simulink library "tether002_ul"  (R2020a)
settings: Solver=VariableStepAuto  StartTime=0.0  StopTime=10.0  RelTol=1e-3
values from neighbouring files (symbols this model uses):
  initNodePos = [INITIALLINE;INITIALLINE;INITIALLINE]    [tether002_ts.m]
  initNodeVel = [zeros(1,numNodes-2);zeros(1,numNodes-2);zeros(1,numNodes-2)]    [tether002_ts.m]
  numNodes = 11    [tether002_ts.m]
undefined symbols (not defined in the file or in its folder): TotoalNodes
libraries: powerlib_meascontrol x11, nodePosToLinkPos_ul x6, dspmtrx3 x4, sharedtransform x3, simulink_extras x2
(part 1 of 4)
settings Model: Creator=mitch  LastModifiedBy=mr-jo

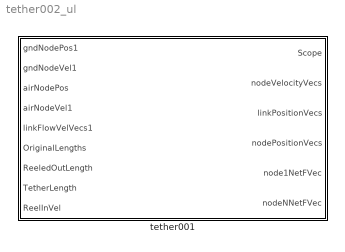
== system tether002_ul ==
  tether001 : Subsystem

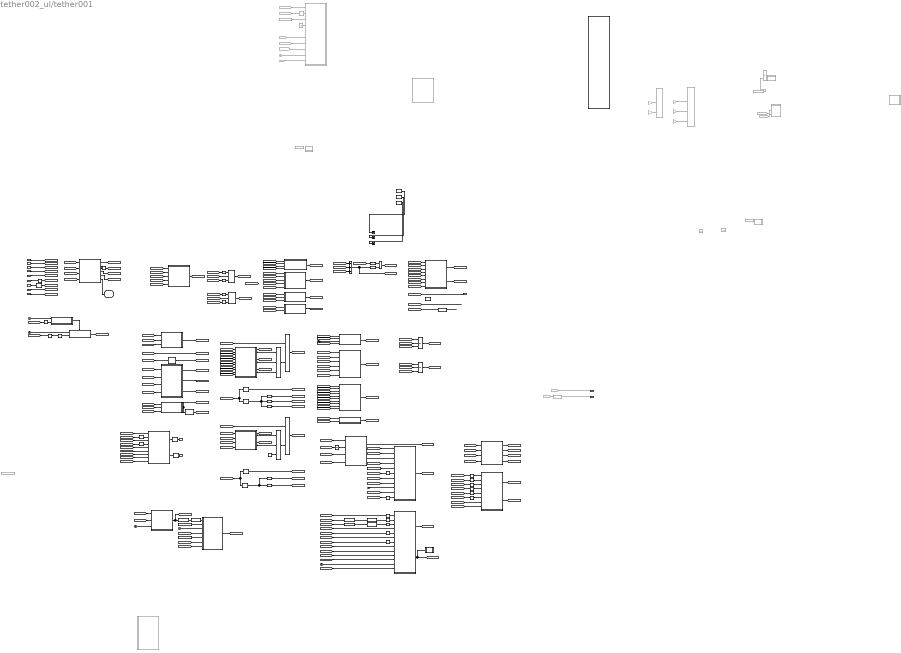
== system tether002_ul/tether001 ==
  note: "Dumbell" Edit
  gndNodePos1 : Inport
  gndNodeVel1 : Inport  Port=2
  airNodePos : Inport  Port=3
  airNodeVel1 : Inport  Port=4
  linkFlowVelVecs1 : Inport  Port=5
  OriginalLengths : Inport  Port=6
  ReeledOutLength : Inport  Port=7
  TetherLength : Inport  Port=8
  ReelInVel : Inport  Port=9
  Add4 : Sum  Inputs=3
  Clock{,1..2,4..7} (7 alike) : Clock
  Clock3 : Clock  Commented=on
  Constant : Constant  Value=0
  Constant1 : Constant  Commented=on  Value=[initNodeVel]
  Constant11 : Constant  Commented=on  Value=[initNodeVel,zeros(3,3)]
  Constant16 : Constant  Value=[initNodeVel,zeros(3,1)]
  Constant2 : Constant  Value=[initNodePos]
  Constant3 : Constant  Value=[numNodes]
  Constant7 : Constant  Commented=on  Value=[initNodePos]
  Direction Cosine Matrix to Rotation Angles : sharedtransform/Direction Cosine Matrix to Rotation Angles  rotationOrder=ZYX  aMode=aMode  action=None  tolerance=eps(2)
      settings: SourceProductBaseCode=AE,PW,MT,VE,VP
  Direction Cosine Matrix to Rotation Angles1 : sharedtransform/Direction Cosine Matrix to Rotation Angles  rotationOrder=ZYX  aMode=aMode  action=None  tolerance=eps(2)
      settings: SourceProductBaseCode=AE,PW,MT,VE,VP
  Direction Cosine Matrix to Rotation Angles2 : sharedtransform/Direction Cosine Matrix to Rotation Angles  rotationOrder=ZYX  aMode=aMode  action=None  tolerance=eps(2)
      settings: SourceProductBaseCode=AE,PW,MT,VE,VP
  First-Order Filter : powerlib_meascontrol/Filters/First-Order Filter  FilterType=Lowpass  Tc=10e-3  Ts=0  Initialize=on  Vac_Init=[0, 0, 60]  Vdc_Init=100  PlotResponse=off  FreqRange="[0,  200,  1]"
  First-Order Filter1 : powerlib_meascontrol/Filters/First-Order Filter  FilterType=Lowpass  Tc=.001  Ts=0  Initialize=on  Vac_Init=[0, 0, 60]  Vdc_Init=0  PlotResponse=off  FreqRange="[0,  200,  1]"
  First-Order Filter{2..4,7..8} (5 alike) : powerlib_meascontrol/Filters/First-Order Filter  FilterType=Lowpass  Tc=1  Ts=0  Initialize=on  Vac_Init=[0, 0, 60]  Vdc_Init=0  PlotResponse=off  FreqRange="[0,  200,  1]"
  First-Order Filter5 : powerlib_meascontrol/Filters/First-Order Filter  FilterType=Lowpass  Tc=10e-3  Ts=0  Initialize=on  Vac_Init=[0, 0, 60]  Vdc_Init=0  PlotResponse=off  FreqRange="[0,  200,  1]"
  First-Order Filter6 : powerlib_meascontrol/Filters/First-Order Filter  FilterType=Lowpass  Tc=10e-3  Ts=0  Initialize=on  Vac_Init=[0, 0, 60]  Vdc_Init=0  PlotResponse=off  FreqRange="[0,  200,  1]"
  From{1,105..106,113} (4 alike) : From  Commented=on  GotoTag=ActiveNodes
  From112 : From  Commented=on  GotoTag=gndNodePos
  From114 : From  Commented=on  GotoTag=OriginalLengths
  From119 : From  Commented=on  GotoTag=Ld
  From161 : From  Commented=on  GotoTag=nodeVel
  From165 : From  Commented=on  GotoTag=nodePos
  From27 : From  Commented=on  GotoTag=o_a_AO_O
  HowManyActive3 : MATLAB Function  TreatAsAtomicUnit=on
  Integrator1 : Integrator  ExternalReset=rising  InitialConditionSource=external
  Integrator8 : Integrator  ExternalReset=rising  InitialConditionSource=external
  Integrator9 : Integrator  Commented=on  InitialConditionSource=external
  MATLAB Function : MATLAB Function  Commented=on  TreatAsAtomicUnit=on
  MATLAB Function1 : MATLAB Function  Commented=on  TreatAsAtomicUnit=on
  MATLAB Function11 : MATLAB Function  Commented=on  TreatAsAtomicUnit=on
  MATLAB Function15 : MATLAB Function  Commented=on  TreatAsAtomicUnit=on
  MATLAB Function2 : MATLAB Function  TreatAsAtomicUnit=on
  MATLAB Function23 : MATLAB Function  TreatAsAtomicUnit=on
  MATLAB Function24 : MATLAB Function  TreatAsAtomicUnit=on
  MATLAB Function25 : MATLAB Function  TreatAsAtomicUnit=on
  MATLAB Function26 : MATLAB Function  Commented=on  TreatAsAtomicUnit=on
  MATLAB Function3 : MATLAB Function  TreatAsAtomicUnit=on
  MATLAB Function34 : MATLAB Function  Commented=on  TreatAsAtomicUnit=on
  MATLAB Function36 : MATLAB Function  TreatAsAtomicUnit=on
  MATLAB Function37 : MATLAB Function  TreatAsAtomicUnit=on
  MATLAB Function38 : MATLAB Function  TreatAsAtomicUnit=on
  MATLAB Function39 : MATLAB Function  TreatAsAtomicUnit=on
  MATLAB Function4 : MATLAB Function  TreatAsAtomicUnit=on
  MATLAB Function40 : MATLAB Function  TreatAsAtomicUnit=on
  MATLAB Function41 : MATLAB Function  TreatAsAtomicUnit=on
  MATLAB Function42 : MATLAB Function  TreatAsAtomicUnit=on
  MATLAB Function43 : MATLAB Function  TreatAsAtomicUnit=on
  MATLAB Function44 : MATLAB Function  TreatAsAtomicUnit=on
  MATLAB Function45 : MATLAB Function  TreatAsAtomicUnit=on
  MATLAB Function46 : MATLAB Function  TreatAsAtomicUnit=on
  MATLAB Function47 : MATLAB Function  TreatAsAtomicUnit=on
  MATLAB Function48 : MATLAB Function  TreatAsAtomicUnit=on
  MATLAB Function49 : MATLAB Function  TreatAsAtomicUnit=on
  MATLAB Function5 : MATLAB Function  TreatAsAtomicUnit=on
  MATLAB Function50 : MATLAB Function  TreatAsAtomicUnit=on
  MATLAB Function51 : MATLAB Function  TreatAsAtomicUnit=on
  MATLAB Function52 : MATLAB Function  TreatAsAtomicUnit=on
  MATLAB Function53 : MATLAB Function  TreatAsAtomicUnit=on
  MATLAB Function6 : MATLAB Function  TreatAsAtomicUnit=on
  MATLAB Function7 : MATLAB Function  Commented=on  TreatAsAtomicUnit=on
  Matrix Concatenate1 : Concatenate  Commented=on  NumInputs=4  Mode=Multidimensional array  ConcatenateDimension=2
  Matrix Concatenate10 : Concatenate  NumInputs=3
  Matrix Concatenate11 : Concatenate  Mode=Multidimensional array  ConcatenateDimension=2
  Matrix Concatenate12 : Concatenate  NumInputs=3  Mode=Multidimensional array  ConcatenateDimension=2
  Matrix Concatenate13 : Concatenate  NumInputs=3  Mode=Multidimensional array  ConcatenateDimension=2
  Matrix Concatenate2 : Concatenate  Commented=on  NumInputs=3  Mode=Multidimensional array  ConcatenateDimension=2
  Matrix Concatenate8 : Concatenate  NumInputs=3
  Matrix Concatenate9 : Concatenate  Mode=Multidimensional array  ConcatenateDimension=2
  Memory{,1..15} (16 alike) : Memory
  Multiply{,1..3,5} (5 alike) : Gain  Commented=on  Gain=[1;1;1]  Multiplication=Matrix(K*u)
  Multiply4 : Product
  Position Reset1 : MATLAB Function  TreatAsAtomicUnit=on
  Position Reset2 : MATLAB Function  Commented=on  TreatAsAtomicUnit=on
  Reshape{31..32,37..38} (4 alike) : Reshape  OutputDimensionality=Column vector (2-D)
  Reshape35 : Reshape  OutputDimensionality=Row vector (2-D)
  Reshape36 : Reshape  OutputDimensionality=Row vector (2-D)
  Selector16 : Selector  NumberOfDimensions=2  InputPortWidth=3  IndexOptions=Index vector (dialog),Index vector (dialog)  Indices=2,1  OutputSizes=1,1
  Selector17 : Selector  NumberOfDimensions=2  InputPortWidth=3  IndexOptions=Index vector (dialog),Index vector (dialog)  Indices=1,1  OutputSizes=1,1
  Selector18 : Selector  NumberOfDimensions=2  InputPortWidth=3  IndexOptions=Select all,Index vector (dialog)  Indices=[1 3],2:numNodes-1  OutputSizes=1,1
  Selector19 : Selector  NumberOfDimensions=2  InputPortWidth=3  IndexOptions=Select all,Index vector (dialog)  Indices=[1 3],2:numNodes-1  OutputSizes=1,1
  Selector20 : Selector  NumberOfDimensions=2  InputPortWidth=1  IndexOptions=Index vector (dialog),Index vector (dialog)  Indices=2,1  OutputSizes=1,1
  Selector21 : Selector  NumberOfDimensions=2  InputPortWidth=1  IndexOptions=Index vector (dialog),Index vector (dialog)  Indices=2,1  OutputSizes=1,1
  Selector22 : Selector  NumberOfDimensions=2  InputPortWidth=3  IndexOptions=Index vector (dialog),Index vector (dialog)  Indices=3,1  OutputSizes=1,1
  Signal Specification : SignalSpecification  Commented=on
  Signal Specification1 : SignalSpecification  Commented=on
  Submatrix1 : dspmtrx3/Submatrix  RowSpan=All rows  RowStartMode=First  RowStartIndex=1  RowEndMode=Last  RowEndIndex=1  ColSpan=Range of columns  ColStartMode=First  ColStartIndex=2  ColEndMode=Index  ColEndIndex=numNodes-2
  Submatrix2 : dspmtrx3/Submatrix  RowSpan=All rows  RowStartMode=First  RowStartIndex=1  RowEndMode=Last  RowEndIndex=1  ColSpan=Range of columns  ColStartMode=Index  ColStartIndex=numNodes-1  ColEndMode=Index  ColEndIndex=numNodes-1
  Submatrix5 : dspmtrx3/Submatrix  RowSpan=All rows  RowStartMode=First  RowStartIndex=1  RowEndMode=Last  RowEndIndex=1  ColSpan=Range of columns  ColStartMode=First  ColStartIndex=2  ColEndMode=Index  ColEndIndex=numNodes-2
  Submatrix6 : dspmtrx3/Submatrix  RowSpan=All rows  RowStartMode=First  RowStartIndex=1  RowEndMode=Last  RowEndIndex=1  ColSpan=Range of columns  ColStartMode=Index  ColStartIndex=numNodes-1  ColEndMode=Index  ColEndIndex=numNodes-1
  Subsystem1 : Subsystem
  Switched derivative for linearization : simulink_extras/Linearization/Switched derivative for linearization  switchVal=1  derivConst=.001
      settings: SourceProductBaseCode=SL
  Switched derivative for linearization1 : simulink_extras/Linearization/Switched derivative for linearization  switchVal=1  derivConst=.001
      settings: SourceProductBaseCode=SL
  Terminator : Terminator
  Terminator1 : Terminator
  Terminator2 : Terminator
  Triggered Subsystem : Subsystem  TreatAsAtomicUnit=on
  Unit Delay{12..14,18} (4 alike) : UnitDelay  Commented=on  SampleTime=-1  HasFrameUpgradeWarning=on
  Unit Delay4 : UnitDelay  SampleTime=-1  HasFrameUpgradeWarning=on
  Velocity Reset1 : MATLAB Function  TreatAsAtomicUnit=on
  nodePosToLinkPos1 : nodePosToLinkPos_ul/nodePosToLinkPos  SystemSampleTime=-1  Latency=0  AutoFrameSizeCalculation=off
  nodePosToLinkPos4 : nodePosToLinkPos_ul/nodePosToLinkPos  Commented=on  SystemSampleTime=-1  Latency=0  AutoFrameSizeCalculation=off
  Scope : Outport  VectorParamsAs1DForOutWhenUnconnected=off
  nodeVelocityVecs : Outport  Port=2  VectorParamsAs1DForOutWhenUnconnected=off
  linkPositionVecs : Outport  Port=3  VectorParamsAs1DForOutWhenUnconnected=off
  nodePositionVecs : Outport  Port=4  VectorParamsAs1DForOutWhenUnconnected=off
  node1NetFVec : Outport  Port=5  VectorParamsAs1DForOutWhenUnconnected=off
  nodeNNetFVec : Outport  Port=6  VectorParamsAs1DForOutWhenUnconnected=off
  wires:
  From27/1 -> MATLAB Function/2(o_a_AO_O)
  From1/1 -> MATLAB Function/3(ActiveNodes)
  Constant11/1 -> Integrator9/2
  Integrator9/1 -> MATLAB Function7/1(Out)
  Multiply2/1 -> Matrix Concatenate1/2
  Multiply5/1 -> Matrix Concatenate1/4
  Multiply3/1 -> Matrix Concatenate1/3
  Multiply1/1 -> Matrix Concatenate2/3
  Multiply/1 -> Matrix Concatenate2/2
  From165/1 -> nodePosToLinkPos4/1
  From161/1 -> nodeVelocityVecs/1  "nodeVelocities"
  nodePosToLinkPos4/1 -> linkPositionVecs/1  "linkPositions"
  Signal Specification/1 -> MATLAB Function15/1(u)
  Unit Delay14/1 -> Position Reset2/2(PrevStepNumNodes)
  From114/1 -> Position Reset2/8(OriginalLengths)
  Clock3/1 -> Position Reset2/9(time)
  From113/1 -> Position Reset2/7(ActiveNodes)
  From112/1 -> Position Reset2/6(gndNodePos)
  From105/1 -> Position Reset2/1(CurStepNumNodes)
  From119/1 -> Position Reset2/10(Ld)
  From106/1 -> Unit Delay14/1
  Constant7/1 -> Position Reset2/3(GivenInit_Pos)
  Unit Delay18/1 -> Position Reset2/4(Previous_Pos)
  [invNodeMasses] -> MATLAB Function47/1(invNodeMasses)
  MATLAB Function39/1(nodeForceVecs) -> [FNetTen]
  Memory3/1 -> MATLAB Function25/3(PosPrevious)
  MATLAB Function53/2(O_c_B_NextNode) -> [O_c_B_NextNode]
  [ActiveNodes] -> Memory7/1
  Integrator8/1 -> [VelocitiesOUT]
  First-Order Filter6/1 -> MATLAB Function37/4(o_a_AO_O)
  [Wy] -> MATLAB Function23/1(Wy)
  MATLAB Function23/1(Theta_dot) -> [Theta_dot], Matrix Concatenate10/1
  MATLAB Function25/2(o_v_AOPrev) -> [o_v_AOPrev]
  Velocity Reset1/2(Vo) -> MATLAB Function52/3("Vo ")
  Unit Delay4/1 -> Velocity Reset1/2(Previous)
  [ReelInVel] -> [Ld]  "Ld"
  [OriginalLengths] -> HowManyActive3/1(OriginalLengths)
  Direction Cosine Matrix to Rotation Angles/1 -> MATLAB Function24/1(R)
  Submatrix2/1 -> Selector22/1, Selector21/1, Selector20/1
  [Psi] -> MATLAB Function49/11(Psi)
  [ActiveNodes] -> Position Reset1/4(CurStepNumNodes)
  Switched derivative for linearization1/1 -> [Ldd]  "Ldd"
  [ActiveLengths] -> Position Reset1/8(ActiveLengths)
  [OriginalLengths] -> Position Reset1/11(OriginalLengths)
  [gndNodeVel] -> Velocity Reset1/3(gndNodeVel)
  [gndNodeVel] -> Reshape38/1
  [FNetTen] -> Add4/2
  [Mad] -> MATLAB Function49/9(Mad)
  Position Reset1/2(Init_Pos_Angle) -> MATLAB Function6/1(u), [PositionIC]
  MATLAB Function23/2(Psi_dot) -> [Psi_dot], Matrix Concatenate10/2
  [ActiveNodes] -> MATLAB Function53/3(ActiveNodes)
  HowManyActive3/3(OriginalNodes) -> [OriginalNodes]
  Memory2/1 -> MATLAB Function25/4(VelPrevious)
  [Wz] -> MATLAB Function44/6(Wz)
  HowManyActive3/1(ActiveNodes) -> [ActiveNodes]
  [nodeVel] -> MATLAB Function41/2(nodeVelocities)
  MATLAB Function53/1(O_c_A_CurrentNode) -> [O_c_A_CurrentNode]
  [Accelerations] -> Integrator8/1
  Submatrix1/1 -> [NodeVelocities]
  [OriginalLengths] -> MATLAB Function52/8(OriginalLengths)
  Memory12/1 -> MATLAB Function52/6(VelocityPrevious)
  [ActiveNodes] -> Position Reset1/10(ActiveNodes)
  [VelecotiesForIntegration] -> Integrator1/1
  [ActiveLengths] -> MATLAB Function52/4(ActiveLengths)
  Memory11/1 -> MATLAB Function52/11(o_v_AOPrev)
  [VelocityBoolean] -> Integrator8/2
  [PositionIC] -> Integrator1/3
  MATLAB Function38/1(A_c_O) -> [A_c_O]
  Selector19/1 -> Multiply4/1
  Selector18/1 -> Multiply4/2
  [O_c_B_NextNode] -> Memory1/1
  Reshape31/1 -> Matrix Concatenate12/1
  gndNodePos1/1 -> [gndNodePos]
  [nodeVel] -> MATLAB Function39/3(nodeVel)
  Memory9/1 -> Position Reset1/2(anglesNext)
  [Wyd] -> MATLAB Function44/5(Wyd)
  MATLAB Function43/1(midNodePosInternal) -> [midNodePosInternal]
  nodePosToLinkPos1/1 -> ?  "linkPositions"
  [NodeVelocities] -> MATLAB Function48/2(VelTotal)
  Matrix Concatenate9/1 -> [Accelerations]
  [Fz] -> MATLAB Function49/7(Fz)
  airNodePos/1 -> [airNodePos]
  gndNodeVel1/1 -> [gndNodeVel]
  [ActiveLengths] -> MATLAB Function40/1(Activelength)
  Memory10/1 -> Position Reset1/1(r_AOPrev)
  [Ld] -> MATLAB Function52/10(Ld)
  Position Reset1/1(Bool) -> [PositionBoolean]
  Memory6/1 -> Position Reset1/7(Previous_Pos_Angle)
  [airNodePos] -> MATLAB Function43/5(airNodePos)
  [Ld] -> Position Reset1/13(Ld)
  [A_c_O] -> MATLAB Function44/1(A_c_O)
  [nodePos] -> MATLAB Function41/1(nodePositions)
  [O_c_A_CurrentNode] -> Direction Cosine Matrix to Rotation Angles2/1
  HowManyActive3/2(ActiveLengths) -> Reshape35/1
  [Ld] -> MATLAB Function44/9(Ld)
  Constant/1 -> Matrix Concatenate10/3
  [gndNodePos] -> Position Reset1/9(gndNodePos)
  [Ld] -> MATLAB Function51/6(Ld)
  [NodeVelocities] -> Matrix Concatenate11/1
  Switched derivative for linearization/1 -> [Mad]
  [NodePositions] -> Memory3/1
  [NodeVelocities] -> Memory2/1
  [ActiveNodes] -> Unit Delay4/1
  [ActiveNodes] -> MATLAB Function25/7(ActiveNodes)
  [Psi] -> MATLAB Function38/2(Psi)
  [Theta_dot] -> MATLAB Function49/1(Theta_dot)
  [PositionsOUT] -> Memory6/1
  Submatrix5/1 -> [NodePositions]
  Memory8/1 -> Position Reset1/3(anglesPrev)
  Matrix Concatenate11/1 -> [VelecotiesForIntegration]
  [o_a_AO_O] -> First-Order Filter6/1
  [airNodePos] -> Reshape37/1
  OriginalLengths/1 -> Reshape36/1
  [invNodeMasses] -> Selector19/1
  [Fx] -> MATLAB Function37/5(Fx)
  Matrix Concatenate13/1 -> [nodeVel]
  [ActiveNodes] -> MATLAB Function45/2(ActiveNodes)
  Reshape38/1 -> Matrix Concatenate13/1
  [ActiveNodes] -> MATLAB Function46/2(ActiveNodes)
  [midNodePos] -> MATLAB Function43/2(midNodePos)
  MATLAB Function51/1(o_v_AO_O) -> [o_v_AO_O]
  [ReelInVel] -> Switched derivative for linearization1/1
  [Wy] -> MATLAB Function44/4(Wy)
  [L] -> MATLAB Function49/3(L)
  [Ldd] -> MATLAB Function44/10(Ldd)
  [nodePos] -> nodePosToLinkPos1/1
  [FNetBuoy] -> Add4/3
  [ActiveNodes] -> MATLAB Function47/3(ActiveNodes)
  [Forces] -> MATLAB Function46/3(Forces)
  [airNodeVel] -> Reshape32/1
  [Wz] -> MATLAB Function23/2(Wz)
  [Ma] -> MATLAB Function49/8(Ma)
  [ActiveNodes] -> Velocity Reset1/1(Current)
  [Wzd] -> MATLAB Function44/7(Wzd)
  MATLAB Function49/3(Wzd) -> [Wzd], Matrix Concatenate8/3
  [gndNodePos] -> MATLAB Function2/1(gndNodePos)
  [Fx] -> MATLAB Function49/5(Fx)
  Submatrix6/1 -> Selector16/1, Selector17/1
  [W_Prev] -> MATLAB Function52/1(W_Prev)
  MATLAB Function49/2(Wyd) -> [Wyd], Matrix Concatenate8/2
  [r_AO_O] -> MATLAB Function48/5(r_AO_O)
  MATLAB Function49/1(Wxd) -> [Wxd], Matrix Concatenate8/1
  Selector22/1 -> [Wz]
  [ActiveLengths] -> MATLAB Function43/4(ActiveLengths)
  [Forces] -> MATLAB Function37/8(Forces)
  Constant16/1 -> MATLAB Function52/5(initNodeVel)
  Selector20/1 -> [Wx]
  [Wx] -> MATLAB Function51/2(Wx)
  airNodeVel1/1 -> [airNodeVel]
  [Wy] -> MATLAB Function51/3(Wy)
  [Theta] -> MATLAB Function49/10(Theta)
  [L] -> MATLAB Function23/4(L)
  Selector17/1 -> [Theta]
  MATLAB Function41/1(nodeForceVecs) -> [FDrag]
  Selector16/1 -> [Psi]
  [Fz] -> MATLAB Function37/7(Fz)
  [Fy] -> MATLAB Function49/6(Fy)
  [gndNodePos] -> MATLAB Function43/1(gndNodePos)
  Direction Cosine Matrix to Rotation Angles2/1 -> MATLAB Function36/1(R)
  Matrix Concatenate12/1 -> [nodePos]
  [TetherLength] -> HowManyActive3/3(TetherLength)
  [VelocityBoolean] -> MATLAB Function52/2(Bool)
  [o_v_AOPrev] -> Memory11/1
  [airNodePos] -> MATLAB Function53/4(airNodePos)
  [OriginalLengths] -> MATLAB Function47/2(OriginalLengths)
  [Mad] -> MATLAB Function37/1(Mad)
  Matrix Concatenate10/1 -> Matrix Concatenate11/2
  [VelocitiesOUT] -> Submatrix1/1, Submatrix2/1
  MATLAB Function47/1(Ma) -> [Ma], Switched derivative for linearization/1
  [L] -> MATLAB Function44/8(L)
  First-Order Filter5/1 -> MATLAB Function37/2(o_v_AO_O)
  [ActiveLengths] -> MATLAB Function25/8(ActiveLengths)
  [OriginalLengths] -> MATLAB Function48/3(OriginalLengths)
  [VelocitiesOUT] -> Memory12/1
  MATLAB Function46/1(Fx) -> [Fx]
  Clock/1 -> Position Reset1/12(time)
  Add4/1 -> [Forces], Selector18/1
  [Theta] -> MATLAB Function38/1(Theta)
  [Fy] -> MATLAB Function37/6(Fy)
  Clock1/1 -> MATLAB Function52/9(time)
  MATLAB Function48/2(midNodeVel) -> [midNodeVel]
  Integrator1/1 -> [PositionsOUT]
  [L] -> MATLAB Function51/5(L)
  [Wz] -> MATLAB Function51/4(Wz)
  Selector21/1 -> [Wy]
  [airNodePos] -> MATLAB Function2/2(airNodePos)
  [Psi_dot] -> MATLAB Function49/2(Psi_dot)
  MATLAB Function52/1(Vo) -> [VelocityIC]
  [ActiveNodes] -> MATLAB Function41/4(NumberNodesActive)
  Reshape35/1 -> [ActiveLengths]
  [ActiveLengths] -> Velocity Reset1/4(ActiveLengths)
  MATLAB Function50/1(r_AO_O) -> [r_AO_O]
  [gndNodePos] -> Reshape31/1
  [ReeledOutLength] -> MATLAB Function39/1(ReeledOutLength)
  [o_v_AO_O] -> First-Order Filter5/1
  [Wxd] -> MATLAB Function44/3(Wxd)
  [o_v_AO_O] -> MATLAB Function48/6(o_v_AO_O)
  [ActiveNodes] -> MATLAB Function48/4(ActiveNodes)
  MATLAB Function25/1(W_Prev) -> [W_Prev]
  [Ma] -> MATLAB Function37/3(Ma)
  Velocity Reset1/1(Bool) -> [VelocityBoolean]
  [NodePositions] -> MATLAB Function48/1(PosTotal)
  [nodePos] -> MATLAB Function42/1(nodePositions)
  [gndNodePos] -> MATLAB Function53/1(gndNodePos)
  [ActiveNodes] -> MATLAB Function52/7(ActiveNodes)
  MATLAB Function45/1(L) -> [L]
  [ActiveNodes] -> MATLAB Function43/3(ActiveNodes)
  [OriginalLengths] -> MATLAB Function45/1(OriginalLengths)
  [r_AO] -> Memory10/1
  ReelInVel/1 -> [ReelInVel]
  [ActiveLengths] -> MATLAB Function45/3(ActiveLengths)
  MATLAB Function40/1(invNodeMasses) -> [invNodeMasses]
  MATLAB Function46/3(Fz) -> [Fz]
  [Ld] -> MATLAB Function49/4(Ld)
  [L] -> MATLAB Function50/2(L)
  [ReeledOutLength] -> HowManyActive3/2(ReeledOutLength)
  TetherLength/1 -> [TetherLength]
  [FDrag] -> Add4/1
  MATLAB Function42/1(nodeForceVecs) -> [FNetBuoy]
  [Wx] -> MATLAB Function44/2(Wx)
  [O_c_A_CurrentNode] -> Memory/1
  [midNodeVel] -> Matrix Concatenate13/2
  [Theta] -> MATLAB Function23/3(Theta)
  [linkFlowVelVecs] -> MATLAB Function41/3(flowVel)
  Reshape32/1 -> Matrix Concatenate13/3
  [PositionsOUT] -> Submatrix5/1, Submatrix6/1
  MATLAB Function46/2(Fy) -> [Fy]
  [O_c_B_NextNode] -> Direction Cosine Matrix to Rotation Angles/1
  Reshape37/1 -> Matrix Concatenate12/3
  Reshape36/1 -> [OriginalLengths]
  Memory/1 -> MATLAB Function25/6(O_c_A_CurrentNode)
  [OriginalLengths] -> MATLAB Function46/1(OriginalLengths)
  linkFlowVelVecs1/1 -> [linkFlowVelVecs]
  MATLAB Function36/1(angles) -> Memory8/1
  MATLAB Function5/1(Given_Pos_Angle_IC) -> [Given_Pos_Angle_IC]
  [VelocityBoolean] -> MATLAB Function46/4(BoolVel)
  [midNodePosInternal] -> Matrix Concatenate12/2
  [A_c_O] -> MATLAB Function51/1(A_c_O)
  MATLAB Function53/4(r_BA) -> [r_BA]
  [nodeVel] -> ?  "nodeVelocities"
  MATLAB Function44/1(o_a_AO_O) -> [o_a_AO_O]
  [midNodePos] -> MATLAB Function53/2(midNodePos)
  [nodePos] -> MATLAB Function39/2(nodePos)
  [NodeAccelerations] -> Matrix Concatenate9/1
  [A_c_O] -> MATLAB Function50/1(A_c_O)
  MATLAB Function48/1(midNodePos) -> [midNodePos]
  Multiply4/1 -> [NodeAccelerations]
  Matrix Concatenate8/1 -> Matrix Concatenate9/2
  [airNodePos] -> Memory5/1
  Memory5/1 -> MATLAB Function25/1(airNodePos)
  [airNodeVel] -> Memory4/1
  Memory4/1 -> MATLAB Function25/2(airNodeVel)
  [gndNodePos] -> MATLAB Function48/7(gndNodePos)
  [gndNodeVel] -> MATLAB Function48/8(gndNodeVel)
  First-Order Filter2/1 -> Terminator/1
  First-Order Filter7/1 -> Terminator1/1
  First-Order Filter8/1 -> Terminator2/1
  Memory1/1 -> MATLAB Function25/5(O_c_B_NextNode)
  Memory7/1 -> Position Reset1/5(PrevStepNumNodes)
  MATLAB Function24/1(angles) -> Memory9/1
  MATLAB Function53/3(r_AO) -> [r_AO]
  Clock4/1 -> MATLAB Function3/1(time)
  Memory13/1 -> Memory15/1
  MATLAB Function3/1(BoolOut) -> Triggered Subsystem/Trigger
  [ActiveNodes] -> MATLAB Function39/5(NumberNodesActive)
  Memory14/1 -> MATLAB Function3/2(Bool)
  Clock6/1 -> MATLAB Function2/3(time)
  Direction Cosine Matrix to Rotation Angles1/1 -> MATLAB Function4/1(R)
  MATLAB Function2/1(Air_c_O_CurrentNode) -> [Air_c_O_CurrentNode], Direction Cosine Matrix to Rotation Angles1/1
  MATLAB Function4/1(angles) -> MATLAB Function5/1(angles)
  Constant2/1 -> MATLAB Function5/2(initNodePos)
  Clock7/1 -> MATLAB Function5/3(time)
  [Given_Pos_Angle_IC] -> Position Reset1/6(GivenInit_Pos_Angle)
  [ActiveNodes] -> MATLAB Function5/4(ActiveNodes)
  Constant3/1 -> MATLAB Function5/5(OriginalNodes)
  [gndNodePos] -> MATLAB Function5/6(gndNodePos)
  [airNodePos] -> MATLAB Function5/7(airNodePos)
  [nodePos] -> nodePositionVecs/1  "nodePositions"
  [ActiveNodes] -> MATLAB Function37/9(ActiveNodes)
  MATLAB Function37/2(nodeNNetFVec) -> First-Order Filter4/1
  ReeledOutLength/1 -> First-Order Filter/1
  First-Order Filter/1 -> [ReeledOutLength]
  [r_BA] -> Memory13/1
  [PositionBoolean] -> Memory14/1
  [ActiveLengths] -> MATLAB Function42/2(ActiveLengths)
  [ActiveNodes] -> MATLAB Function40/2(ActiveNodes)
  [ActiveNodes] -> MATLAB Function42/3(NumberNodesActive)
  [Lcorrected] -> HowManyActive3/4(Lcorrected)
  Clock2/1 -> Triggered Subsystem/1(time)
  Clock5/1 -> MATLAB Function50/3(time)
  [Air_c_O_CurrentNode] -> MATLAB Function50/4(Air_c_O_CurrentNode)
  HowManyActive3/4(ActiveLengthsUncorrected) -> [ActiveLengthsUncorrected]
  [ActiveLengthsUncorrected] -> MATLAB Function39/4(ActiveLengths)
  MATLAB Function37/1(node1NetFVec) -> First-Order Filter3/1
  [VelocityIC] -> Integrator8/3
  [PositionBoolean] -> Integrator1/2
  Triggered Subsystem/1(Lcorrected) -> [Lcorrected]
  HowManyActive3/5(Scope) -> Scope/1
  Memory15/1 -> Triggered Subsystem/2(r_BA)
  First-Order Filter3/1 -> node1NetFVec/1
  First-Order Filter4/1 -> nodeNNetFVec/1
